simulink model "figure12"  (R2015b)
settings: Solver=FixedStepAuto  StartTime=0.0  StopTime=10  RelTol=1e-3
values from neighbouring files (symbols this model uses):
  bHI = 35    [Initiation.m]
  kWall = 90000    [Initiation.m]    (also in VirtualEnvironment.m = block.DialogPrm(1).Data; Virtual_Environment.m = block.DialogPrm(1).Data)
  m = 1    [Initiation.m]
  tsampling = 0.001    [Initiation.m]    (also in VirtualEnvironment.m = block.DialogPrm(6).Data; Virtual_Environment.m = block.DialogPrm(6).Data)
  xWall = 0.085    [Initiation.m]
undefined symbols (not defined in the file or in its folder): DiscIntNeverNeededParam
libraries: simulink x1
settings Model: Creator=TOSHIBA  LastModifiedBy=TOSHIBA

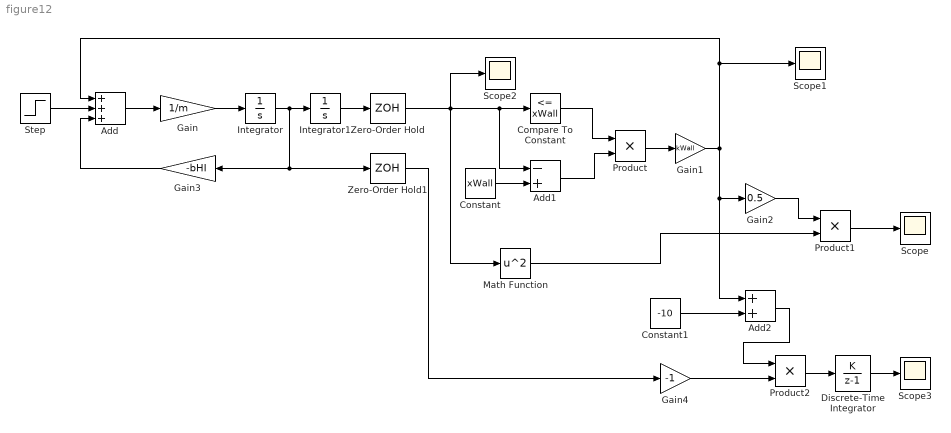
== system figure12 ==
  Add : Sum  Inputs=+++
  Add1 : Sum  Inputs=-+
  Add2 : Sum
  Compare To Constant : simulink/Logic and Bit Operations/Compare To Constant  relop=<=  const=xWall  OutDataTypeStr=boolean
  Constant : Constant  Value=xWall
  Constant1 : Constant  Value=-10
  Discrete-Time Integrator : DiscreteIntegrator  IntegratorMethod=Accumulation: Forward Euler  InitialConditionSetting=State (most efficient)  SampleTime=tsampling  ICPrevOutput=DiscIntNeverNeededParam  ICPrevScaledInput=DiscIntNeverNeededParam
  Gain : Gain  Gain=1/m
  Gain1 : Gain  Gain=kWall
  Gain2 : Gain  Gain=0.5
  Gain3 : Gain  Gain=-bHI
  Gain4 : Gain  Gain=-1
  Integrator : Integrator
  Integrator1 : Integrator  InitialCondition=0.14
  Math Function : Math  Operator=square  SaturateOnIntegerOverflow=on
  Product : Product
  Product1 : Product
  Product2 : Product
  Scope{,1..3} (4 alike) : Scope
  Step : Step  Time=0.35  After=-50  SampleTime=0
  Zero-Order Hold : ZeroOrderHold  SampleTime=tsampling
  Zero-Order Hold1 : ZeroOrderHold  SampleTime=tsampling
  wires:
  Step/1 -> Add/2
  Add/1 -> Gain/1
  Gain/1 -> Integrator/1
  Integrator/1 -> Zero-Order Hold1/1, Gain3/1, Integrator1/1
  Constant/1 -> Add1/2
  Compare To Constant/1 -> Product/1
  Add1/1 -> Product/2
  Product/1 -> Gain1/1
  Gain1/1 -> Add2/1, Gain2/1, Scope1/1, Add/1
  Math Function/1 -> Product1/2
  Product1/1 -> Scope/1
  Integrator1/1 -> Zero-Order Hold/1
  Gain2/1 -> Product1/1
  Gain3/1 -> Add/3
  Zero-Order Hold/1 -> Scope2/1, Math Function/1, Add1/1, Compare To Constant/1
  Zero-Order Hold1/1 -> Gain4/1
  Product2/1 -> Discrete-Time Integrator/1
  Discrete-Time Integrator/1 -> Scope3/1
  Gain4/1 -> Product2/2
  Constant1/1 -> Add2/2
  Add2/1 -> Product2/1
